simulink model "fancyBlinker"  (R2020a)
settings: Solver=ode3  StartTime=0.0  StopTime=inf  FixedStep=.01  RelTol=1e-3  EnableMultiTasking=on
libraries: bbblueSensorLib x1, bbblueBasicLib x1, lab1Library x1
settings Model: SimulationMode=external  ExtModeTrigDuration=100  Creator=Sal  LastModifiedBy=crsmyth
settings SolverCC: PositivePriorityOrder=on  AutoInsertRateTranBlk=on
settings DataIOCC: SaveOperatingPoint=on  SaveFormat=StructureWithTime  ReturnWorkspaceOutputs=off
settings OptimizationCC: EnhancedBackFolding=on  PassReuseOutputArgsAs=Individual arguments  ZeroExternalMemoryAtStartup=off  ZeroInternalMemoryAtStartup=off  MaxStackSize=64  OptimizeBlockOrder=speed  DifferentSizesBufferReuse=on  OptimizationCustomize=off  EfficientTunableParamExpr=on
settings DebuggingCC: ParameterTunabilityLossMsg=error
settings HardwareCC: ProdBitPerPointer=32  ProdBitPerSizeT=32  ProdBitPerPtrDiffT=32  ProdLargestAtomicInteger=Long  ProdLargestAtomicFloat=Double  ProdWordSize=32  ProdHWDeviceType=ARM Compatible->ARM Cortex
settings SFSimCC: MATLABDynamicMemAlloc=off
settings RTWCC: SystemTargetFile=ert.tlc  HardwareBoard=BeagleBone Blue  TemplateMakefile=ert_default_tmf  Toolchain=GNU GCC BeagleBone Blue
settings CodeAppCC: ForceParamTrailComments=on  IgnoreCustomStorageClasses=off  OperatorAnnotations=on  SimulinkDataObjDesc=on  SFDataObjDesc=on  InsertBlockDesc=on
settings ERTTargetCC: MatFileLogging=on  SupportContinuousTime=on  SupportVariableSizeSignals=on

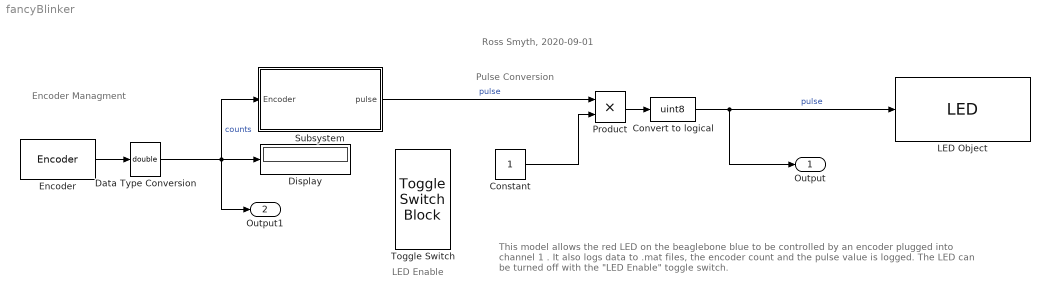
== system fancyBlinker ==
  note: Ross Smyth, 2020-09-01
  note: This model allows the red LED on the beaglebone blue to be controlled by an encoder plugged into channel 1 .
      | It also logs data to .mat files, the encoder count and the pulse value is logged. The LED can be turned off with the "LED Enable"
      | toggle switch.
  note: Pulse Conversion
  note: Encoder Managment
  note: LED
      | Enable
  Constant : Constant
  Convert to logical : DataTypeConversion  OutDataTypeStr=uint8
  Data Type Conversion : DataTypeConversion  OutDataTypeStr=double
  Display : Display
  Encoder : bbblueSensorLib/Encoder  Channel=1  Mode=No reset  SampleTime=0.1  SimulateUsing=Code generation
      settings: SourceProductBaseCode=SC_BEAGLEBONE_BLUE
  LED Object : bbblueBasicLib/LED  LED=Red
      settings: SourceProductBaseCode=SC_BEAGLEBONE_BLUE
  Product : Product
  Subsystem : Subsystem
  Toggle Switch : ToggleSwitchBlock  LabelPosition=Hide
      settings: Values={{'Off', 'On'}, [0 1]}
  Output : Outport
  Output1 : Outport  Port=2
  wires:
  Subsystem/1(pulse) -> Product/1  "pulse"
  Convert to logical/1 -> Output/1, LED Object/1  "pulse"
  Product/1 -> Convert to logical/1
  Constant/1 -> Product/2
  Encoder/1 -> Data Type Conversion/1
  Data Type Conversion/1 -> Subsystem/1(Encoder), Output1/1, Display/1  "counts"

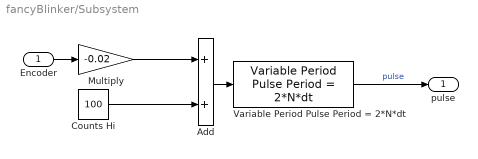
== system fancyBlinker/Subsystem ==
  Encoder : Inport
  Add : Sum
  Counts Hi : Constant  Value=100
  Multiply : Gain  Gain=-0.02
  Variable Period Pulse Period = 2*N*dt : lab1Library/Variable Period Pulse Period = 2*N*dt
  pulse : Outport
  wires:
  Encoder/1 -> Multiply/1
  Variable Period Pulse Period = 2*N*dt/1 -> pulse/1  "pulse"
  Add/1 -> Variable Period Pulse Period = 2*N*dt/1
  Multiply/1 -> Add/1
  Counts Hi/1 -> Add/2
